simulink model "pcssp_KMAG"  (R2021b)
settings: configuration reference "configurationSettings" (kept outside this file)
model workspace (MAT data in the model file):
  D = Simulink.Parameter
  D.Value = [1; 1; 1; 1; 1; 1; 1; 1; 1; 1]
  D.DataType = 'auto'
  D.Complexity = 'real'
  D.Dimensions = [10 1]
  I = Simulink.Parameter
  I.Value = [0; 0; 0; 0; 0; 0; 0; 0; 0; 0]
  I.DataType = 'auto'
  I.Complexity = 'real'
  I.Dimensions = [10 1]
  Ke = Simulink.Parameter
  Ke.Value = [-28670  34910  -109600  -61980  15820  1380  -79930  5000  -33750  107970; -4300  49190  266010  -320680  -89150  -14470  213760  -294110  141230  -69990; -8230  89070  -109150  128070  -98530  23030  -80450  198760  -447440  298310; 60280  -203200  325320  92860  19480  -28160  246550  -127230  418190  -542920; 27220  -53430  89760  38240  33040  -9510  58170  -41770  149520  -165290; -64820  62380  -448030  96250  75680  20610  -335880  248860  -252220  351720; -79530  20450  -526450  190300  68090  33330  -374430  359300  -304180  362660; -14110  -195650  264260  12300  -144100  28740  302600  -17230  198910  -331740; 31190  108560  160080  -115050  -57970  36320  136890  -80820  -59420  128610; 16680  216660  -299770  45470  127150  30260  -279790  136410  -267230  459950; 35820  72090  -113700  76140  123830  5400  -131940  47420  -1940  106630]
  Ke.DataType = 'auto'
  Ke.Complexity = 'real'
  Ke.Dimensions = [11 10]
  N = Simulink.Parameter
  N.Value = [100; 100; 100; 100; 100; 100; 100; 100; 100; 100]
  N.DataType = 'auto'
  N.Complexity = 'real'
  N.Dimensions = [10 1]
  P = Simulink.Parameter
  P.Value = [1; 1; 1; 1; 1; 1; 1; 1; 1; 1]
  P.DataType = 'auto'
  P.Complexity = 'real'
  P.Dimensions = [10 1]
values from neighbouring files (symbols this model uses):
  D = Simulink.Parameter(ones(10,1))    [pcssp_KMAG_load_D.m]
  I = Simulink.Parameter(zeros(10,1))    [pcssp_KMAG_load_I.m]
  Ke = Simulink.Parameter(Ketemp)    [pcssp_KMAG_load_Ke.m]
  N = Simulink.Parameter(100*ones(10,1))    [pcssp_KMAG_load_N.m]
  P = Simulink.Parameter(ones(10,1))    [pcssp_KMAG_load_P.m]
  pcssp_KMAG_fp = 0.0    [pcssp_KMAG.sldd]
undefined symbols (not defined in the file or in its folder): DiscIntNeverNeededParam
settings Model: DataDictionary=pcssp_KMAG.sldd  Creator=ravenst1  LastModifiedBy=ravenst1
settings ConfigSetRef: SourceName=configurationSettings

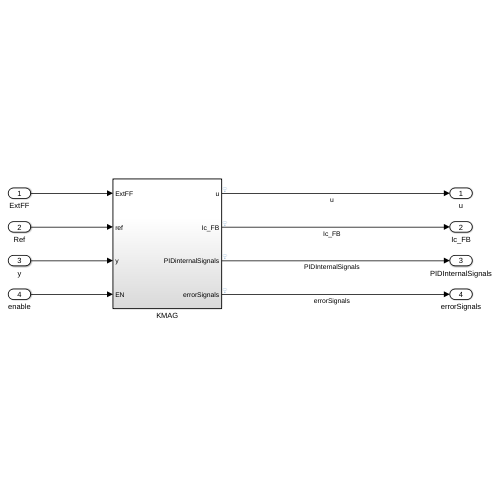
[thumbnail: Simulink's stored preview of the top-level diagram]
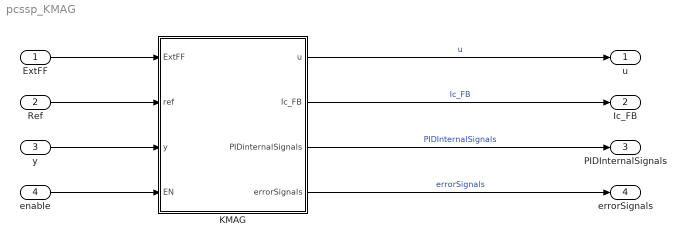
== system pcssp_KMAG ==
  ExtFF : Inport  PortDimensions=size.extFF
  Ref : Inport  Port=2  PortDimensions=size.Ref
  y : Inport  Port=3  PortDimensions=size.y
  enable : Inport  Port=4  OutDataTypeStr=double  PortDimensions=size.enable
  KMAG : Subsystem
  u : Outport
  Ic_FB : Outport  Port=2
  PIDInternalSignals : Outport  Port=3
  errorSignals : Outport  Port=4
  wires:
  KMAG/1(u) -> u/1  "u"
  KMAG/4(errorSignals) -> errorSignals/1  "errorSignals"
  KMAG/3(PIDinternalSignals) -> PIDInternalSignals/1  "PIDInternalSignals"
  KMAG/2(Ic_FB) -> Ic_FB/1  "Ic_FB"
  enable/1 -> KMAG/4(EN)
  ExtFF/1 -> KMAG/1(ExtFF)
  Ref/1 -> KMAG/2(ref)
  y/1 -> KMAG/3(y)

== system pcssp_KMAG/KMAG ==
  ExtFF : Inport
  ref : Inport  Port=2
  y : Inport  Port=3
  EN : Inport  Port=4
  "Enabled PID Block with Enabled Integration (10x10) " : Subsystem
  Ke : Constant  Value=Ke
  Logical Operator : Logic  Operator=NOT  AllPortsSameDT=off  OutDataTypeStr=boolean
  Multiply1 : Product  Inputs=**  Multiplication=Matrix(*)
  Sum : Sum  Inputs=|+-
  Sum1 : Sum  Inputs=++|
  Switch : Switch  Criteria=u2 > Threshold
  ones(10,1) : Constant  Value=1*ones(10,1)
  zeros(10,1) : Constant  Value=0
  u : Outport  PortDimensions=size.extFF
  Ic_FB : Outport  Port=2
  PIDinternalSignals : Outport  Port=3
  errorSignals : Outport  Port=4
  wires:
  "Enabled PID Block with Enabled Integration (10x10) "/1(u) -> Multiply1/2
  Sum1/1 -> Switch/3
  Logical Operator/1 -> Switch/2
  zeros(10,1)/1 -> "Enabled PID Block with Enabled Integration (10x10) "/3(Rs)
  Ke/1 -> Multiply1/1
  Sum/1 -> errorSignals/1, "Enabled PID Block with Enabled Integration (10x10) "/1(e)
  ExtFF/1 -> Sum1/1, Switch/1
  "Enabled PID Block with Enabled Integration (10x10) "/2(PIDinternalSignals) -> PIDinternalSignals/1
  ones(10,1)/1 -> "Enabled PID Block with Enabled Integration (10x10) "/2(IES)
  EN/1 -> Logical Operator/1, "Enabled PID Block with Enabled Integration (10x10) "/Enable
  ref/1 -> Sum/1
  Multiply1/1 -> Sum1/2, Ic_FB/1
  Switch/1 -> u/1
  y/1 -> Sum/2

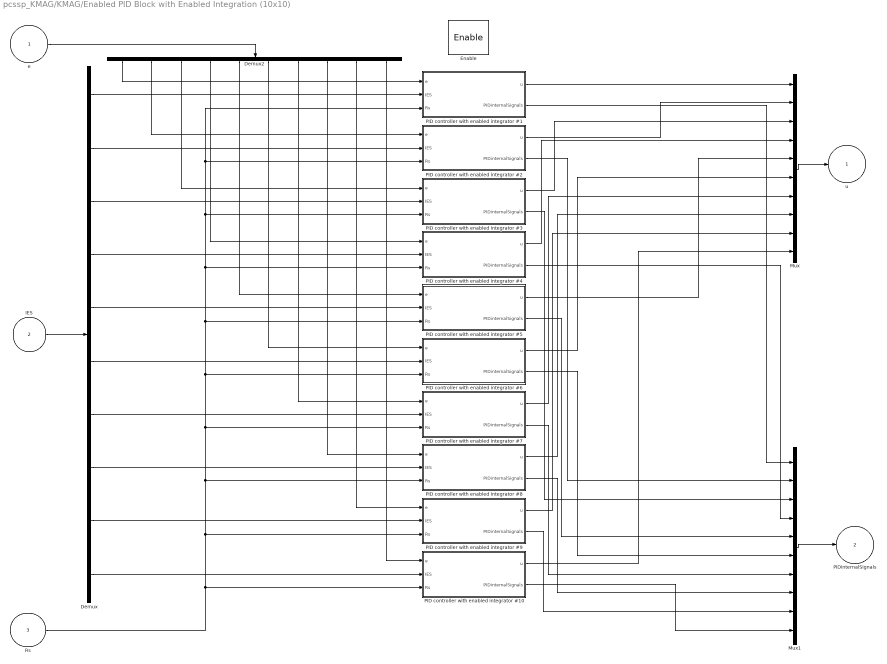
== system pcssp_KMAG/KMAG/Enabled PID Block with Enabled Integration (10x10)  ==
  e : Inport
  IES : Inport  Port=2
  Rs : Inport  Port=3
  Enable : EnablePort  StatesWhenEnabling=reset
  Demux : Demux  Outputs=10
  Demux2 : Demux  Outputs=10
  Mux : Mux  Inputs=10
  Mux1 : Mux  Inputs=10
  PID controller with enabled integrator #1 : Subsystem
  PID controller with enabled integrator #10 : Subsystem
  PID controller with enabled integrator #2 : Subsystem
  PID controller with enabled integrator #3 : Subsystem
  PID controller with enabled integrator #4 : Subsystem
  PID controller with enabled integrator #5 : Subsystem
  PID controller with enabled integrator #6 : Subsystem
  PID controller with enabled integrator #7 : Subsystem
  PID controller with enabled integrator #8 : Subsystem
  PID controller with enabled integrator #9 : Subsystem
  u : Outport
  PIDinternalSignals : Outport  Port=2
  wires:
  e/1 -> Demux2/1
  IES/1 -> Demux/1
  PID controller with enabled integrator #5/2(PIDinternalSignals) -> Mux1/5
  PID controller with enabled integrator #4/2(PIDinternalSignals) -> Mux1/4
  PID controller with enabled integrator #3/2(PIDinternalSignals) -> Mux1/3
  PID controller with enabled integrator #2/2(PIDinternalSignals) -> Mux1/2
  PID controller with enabled integrator #1/2(PIDinternalSignals) -> Mux1/1
  PID controller with enabled integrator #6/2(PIDinternalSignals) -> Mux1/6
  PID controller with enabled integrator #7/2(PIDinternalSignals) -> Mux1/7
  PID controller with enabled integrator #8/2(PIDinternalSignals) -> Mux1/8
  PID controller with enabled integrator #9/2(PIDinternalSignals) -> Mux1/9
  PID controller with enabled integrator #10/2(PIDinternalSignals) -> Mux1/10
  PID controller with enabled integrator #1/1(u) -> Mux/1
  PID controller with enabled integrator #2/1(u) -> Mux/2
  PID controller with enabled integrator #3/1(u) -> Mux/3
  PID controller with enabled integrator #4/1(u) -> Mux/4
  PID controller with enabled integrator #5/1(u) -> Mux/5
  PID controller with enabled integrator #6/1(u) -> Mux/6
  PID controller with enabled integrator #7/1(u) -> Mux/7
  PID controller with enabled integrator #8/1(u) -> Mux/8
  PID controller with enabled integrator #9/1(u) -> Mux/9
  PID controller with enabled integrator #10/1(u) -> Mux/10
  Mux1/1 -> PIDinternalSignals/1
  Demux/4 -> PID controller with enabled integrator #4/2(IES)
  Demux2/9 -> PID controller with enabled integrator #9/1(e)
  Demux/7 -> PID controller with enabled integrator #7/2(IES)
  Rs/1 -> PID controller with enabled integrator #10/3(Rs), PID controller with enabled integrator #9/3(Rs), PID controller with enabled integrator #8/3(Rs), PID controller with enabled integrator #7/3(Rs), PID controller with enabled integrator #6/3(Rs), PID controller with enabled integrator #5/3(Rs), PID controller with enabled integrator #4/3(Rs), PID controller with enabled integrator #3/3(Rs), PID controller with enabled integrator #2/3(Rs), PID controller with enabled integrator #1/3(Rs)
  Demux/1 -> PID controller with enabled integrator #1/2(IES)
  Demux/5 -> PID controller with enabled integrator #5/2(IES)
  Demux/6 -> PID controller with enabled integrator #6/2(IES)
  Demux/2 -> PID controller with enabled integrator #2/2(IES)
  Demux/8 -> PID controller with enabled integrator #8/2(IES)
  Demux/10 -> PID controller with enabled integrator #10/2(IES)
  Demux2/10 -> PID controller with enabled integrator #10/1(e)
  Demux2/4 -> PID controller with enabled integrator #4/1(e)
  Demux2/3 -> PID controller with enabled integrator #3/1(e)
  Demux2/2 -> PID controller with enabled integrator #2/1(e)
  Demux/3 -> PID controller with enabled integrator #3/2(IES)
  Demux2/5 -> PID controller with enabled integrator #5/1(e)
  Mux/1 -> u/1
  Demux2/8 -> PID controller with enabled integrator #8/1(e)
  Demux2/7 -> PID controller with enabled integrator #7/1(e)
  Demux2/6 -> PID controller with enabled integrator #6/1(e)
  Demux/9 -> PID controller with enabled integrator #9/2(IES)
  Demux2/1 -> PID controller with enabled integrator #1/1(e)

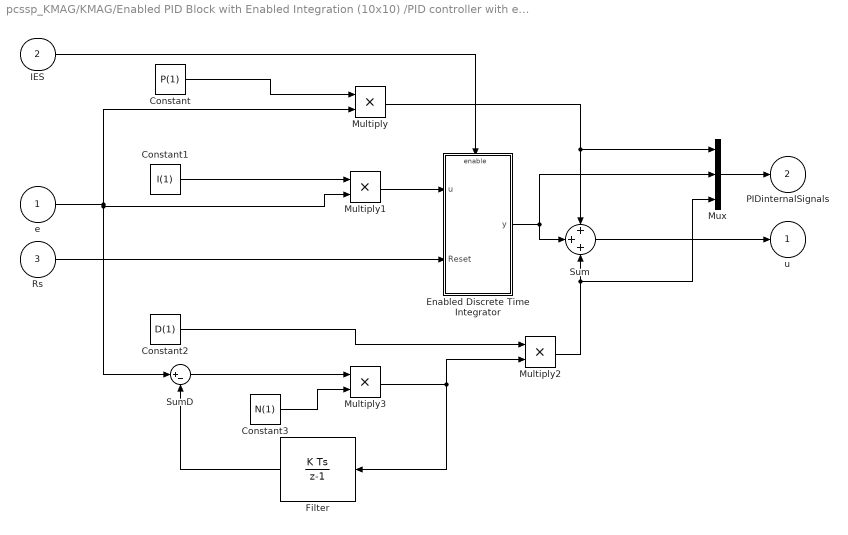
== system pcssp_KMAG/KMAG/Enabled PID Block with Enabled Integration (10x10) /PID controller with enabled integrator #1 ==
  e : Inport
  IES : Inport  Port=2
  Rs : Inport  Port=3
  Constant : Constant  Value=P(1)
  Constant1 : Constant  Value=I(1)
  Constant2 : Constant  Value=D(1)
  Constant3 : Constant  Value=N(1)
  Enabled Discrete Time Integrator : Subsystem
  Filter : DiscreteIntegrator  DisableCoverage=on  SampleTime=pcssp_KMAG_fp.timing.dt  ICPrevOutput=DiscIntNeverNeededParam  ICPrevScaledInput=DiscIntNeverNeededParam
  Multiply{,1..3} (4 alike) : Product  Inputs=**
  Mux : Mux  Inputs=3
  Sum : Sum  Inputs=+++
  SumD : Sum  DisableCoverage=on  Inputs=|+-
  u : Outport  InitialOutput=0
  PIDinternalSignals : Outport  Port=2  InitialOutput=0
  wires:
  Multiply1/1 -> Enabled Discrete Time Integrator/1(u)
  Filter/1 -> SumD/2
  Enabled Discrete Time Integrator/1(y) -> Mux/2, Sum/2
  IES/1 -> Enabled Discrete Time Integrator/Enable
  Sum/1 -> u/1
  Multiply/1 -> Sum/1, Mux/1
  e/1 -> Multiply/2, Multiply1/2, SumD/1
  Rs/1 -> Enabled Discrete Time Integrator/2(Reset)
  Mux/1 -> PIDinternalSignals/1
  Constant/1 -> Multiply/1
  Multiply3/1 -> Multiply2/2, Filter/1
  Constant2/1 -> Multiply2/1
  Multiply2/1 -> Sum/3, Mux/3
  Constant3/1 -> Multiply3/2
  SumD/1 -> Multiply3/1
  Constant1/1 -> Multiply1/1

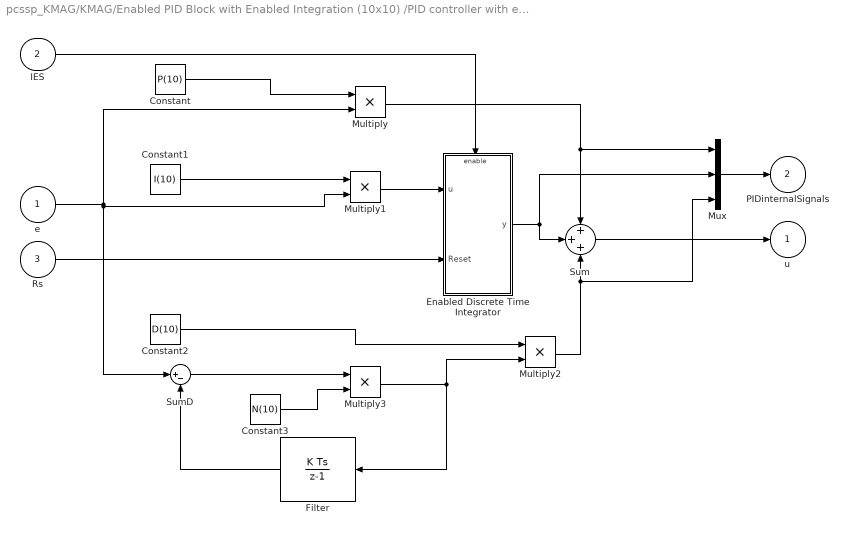
== system pcssp_KMAG/KMAG/Enabled PID Block with Enabled Integration (10x10) /PID controller with enabled integrator #10 ==
  e : Inport
  IES : Inport  Port=2
  Rs : Inport  Port=3
  Constant : Constant  Value=P(10)
  Constant1 : Constant  Value=I(10)
  Constant2 : Constant  Value=D(10)
  Constant3 : Constant  Value=N(10)
  Enabled Discrete Time Integrator : Subsystem
  Filter : DiscreteIntegrator  DisableCoverage=on  SampleTime=pcssp_KMAG_fp.timing.dt  ICPrevOutput=DiscIntNeverNeededParam  ICPrevScaledInput=DiscIntNeverNeededParam
  Multiply{,1..3} (4 alike) : Product  Inputs=**
  Mux : Mux  Inputs=3
  Sum : Sum  Inputs=+++
  SumD : Sum  DisableCoverage=on  Inputs=|+-
  u : Outport  InitialOutput=0
  PIDinternalSignals : Outport  Port=2  InitialOutput=0
  wires:
  Multiply1/1 -> Enabled Discrete Time Integrator/1(u)
  Filter/1 -> SumD/2
  Enabled Discrete Time Integrator/1(y) -> Mux/2, Sum/2
  IES/1 -> Enabled Discrete Time Integrator/Enable
  Sum/1 -> u/1
  Multiply/1 -> Sum/1, Mux/1
  e/1 -> Multiply/2, Multiply1/2, SumD/1
  Rs/1 -> Enabled Discrete Time Integrator/2(Reset)
  Mux/1 -> PIDinternalSignals/1
  Constant/1 -> Multiply/1
  Multiply3/1 -> Multiply2/2, Filter/1
  Constant2/1 -> Multiply2/1
  Multiply2/1 -> Sum/3, Mux/3
  Constant3/1 -> Multiply3/2
  SumD/1 -> Multiply3/1
  Constant1/1 -> Multiply1/1

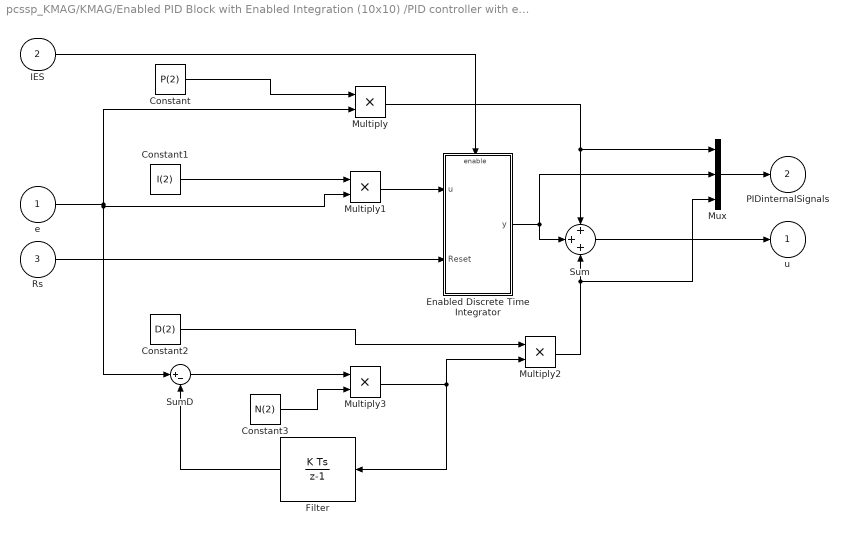
== system pcssp_KMAG/KMAG/Enabled PID Block with Enabled Integration (10x10) /PID controller with enabled integrator #2 ==
  e : Inport
  IES : Inport  Port=2
  Rs : Inport  Port=3
  Constant : Constant  Value=P(2)
  Constant1 : Constant  Value=I(2)
  Constant2 : Constant  Value=D(2)
  Constant3 : Constant  Value=N(2)
  Enabled Discrete Time Integrator : Subsystem
  Filter : DiscreteIntegrator  DisableCoverage=on  SampleTime=pcssp_KMAG_fp.timing.dt  ICPrevOutput=DiscIntNeverNeededParam  ICPrevScaledInput=DiscIntNeverNeededParam
  Multiply{,1..3} (4 alike) : Product  Inputs=**
  Mux : Mux  Inputs=3
  Sum : Sum  Inputs=+++
  SumD : Sum  DisableCoverage=on  Inputs=|+-
  u : Outport  InitialOutput=0
  PIDinternalSignals : Outport  Port=2  InitialOutput=0
  wires:
  Multiply1/1 -> Enabled Discrete Time Integrator/1(u)
  Filter/1 -> SumD/2
  Enabled Discrete Time Integrator/1(y) -> Mux/2, Sum/2
  IES/1 -> Enabled Discrete Time Integrator/Enable
  Sum/1 -> u/1
  Multiply/1 -> Sum/1, Mux/1
  e/1 -> Multiply/2, Multiply1/2, SumD/1
  Rs/1 -> Enabled Discrete Time Integrator/2(Reset)
  Mux/1 -> PIDinternalSignals/1
  Constant/1 -> Multiply/1
  Multiply3/1 -> Multiply2/2, Filter/1
  Constant2/1 -> Multiply2/1
  Multiply2/1 -> Sum/3, Mux/3
  Constant3/1 -> Multiply3/2
  SumD/1 -> Multiply3/1
  Constant1/1 -> Multiply1/1

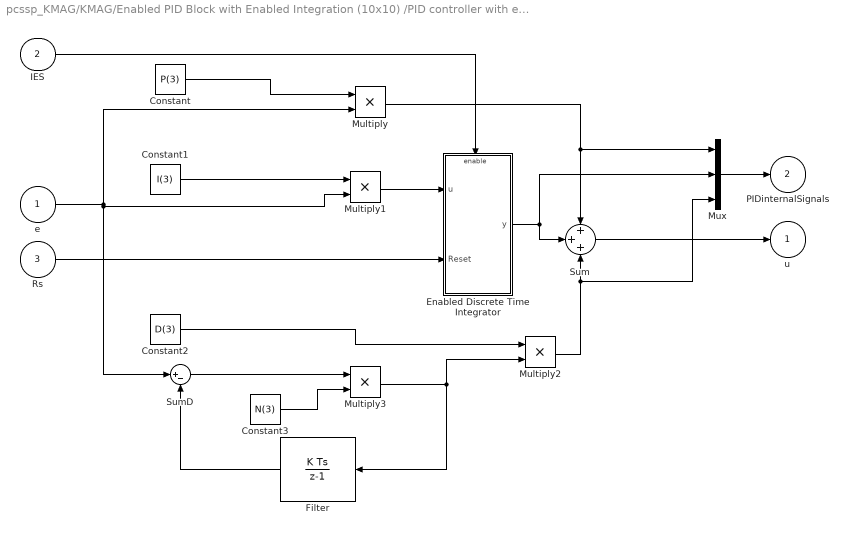
== system pcssp_KMAG/KMAG/Enabled PID Block with Enabled Integration (10x10) /PID controller with enabled integrator #3 ==
  e : Inport
  IES : Inport  Port=2
  Rs : Inport  Port=3
  Constant : Constant  Value=P(3)
  Constant1 : Constant  Value=I(3)
  Constant2 : Constant  Value=D(3)
  Constant3 : Constant  Value=N(3)
  Enabled Discrete Time Integrator : Subsystem
  Filter : DiscreteIntegrator  DisableCoverage=on  SampleTime=pcssp_KMAG_fp.timing.dt  ICPrevOutput=DiscIntNeverNeededParam  ICPrevScaledInput=DiscIntNeverNeededParam
  Multiply{,1..3} (4 alike) : Product  Inputs=**
  Mux : Mux  Inputs=3
  Sum : Sum  Inputs=+++
  SumD : Sum  DisableCoverage=on  Inputs=|+-
  u : Outport  InitialOutput=0
  PIDinternalSignals : Outport  Port=2  InitialOutput=0
  wires:
  Multiply1/1 -> Enabled Discrete Time Integrator/1(u)
  Filter/1 -> SumD/2
  Enabled Discrete Time Integrator/1(y) -> Mux/2, Sum/2
  IES/1 -> Enabled Discrete Time Integrator/Enable
  Sum/1 -> u/1
  Multiply/1 -> Sum/1, Mux/1
  e/1 -> Multiply/2, Multiply1/2, SumD/1
  Rs/1 -> Enabled Discrete Time Integrator/2(Reset)
  Mux/1 -> PIDinternalSignals/1
  Constant/1 -> Multiply/1
  Multiply3/1 -> Multiply2/2, Filter/1
  Constant2/1 -> Multiply2/1
  Multiply2/1 -> Sum/3, Mux/3
  Constant3/1 -> Multiply3/2
  SumD/1 -> Multiply3/1
  Constant1/1 -> Multiply1/1

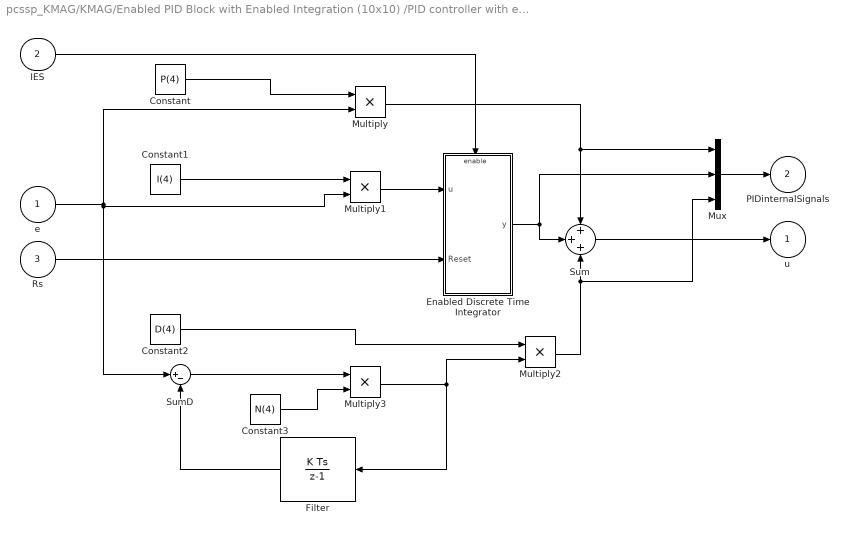
== system pcssp_KMAG/KMAG/Enabled PID Block with Enabled Integration (10x10) /PID controller with enabled integrator #4 ==
  e : Inport
  IES : Inport  Port=2
  Rs : Inport  Port=3
  Constant : Constant  Value=P(4)
  Constant1 : Constant  Value=I(4)
  Constant2 : Constant  Value=D(4)
  Constant3 : Constant  Value=N(4)
  Enabled Discrete Time Integrator : Subsystem
  Filter : DiscreteIntegrator  DisableCoverage=on  SampleTime=pcssp_KMAG_fp.timing.dt  ICPrevOutput=DiscIntNeverNeededParam  ICPrevScaledInput=DiscIntNeverNeededParam
  Multiply{,1..3} (4 alike) : Product  Inputs=**
  Mux : Mux  Inputs=3
  Sum : Sum  Inputs=+++
  SumD : Sum  DisableCoverage=on  Inputs=|+-
  u : Outport  InitialOutput=0
  PIDinternalSignals : Outport  Port=2  InitialOutput=0
  wires:
  Multiply1/1 -> Enabled Discrete Time Integrator/1(u)
  Filter/1 -> SumD/2
  Enabled Discrete Time Integrator/1(y) -> Mux/2, Sum/2
  IES/1 -> Enabled Discrete Time Integrator/Enable
  Sum/1 -> u/1
  Multiply/1 -> Sum/1, Mux/1
  e/1 -> Multiply/2, Multiply1/2, SumD/1
  Rs/1 -> Enabled Discrete Time Integrator/2(Reset)
  Mux/1 -> PIDinternalSignals/1
  Constant/1 -> Multiply/1
  Multiply3/1 -> Multiply2/2, Filter/1
  Constant2/1 -> Multiply2/1
  Multiply2/1 -> Sum/3, Mux/3
  Constant3/1 -> Multiply3/2
  SumD/1 -> Multiply3/1
  Constant1/1 -> Multiply1/1

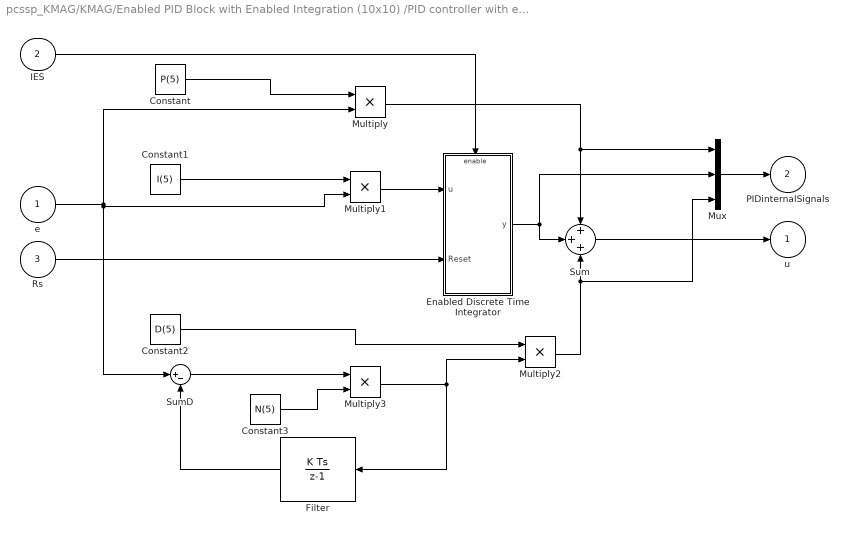
== system pcssp_KMAG/KMAG/Enabled PID Block with Enabled Integration (10x10) /PID controller with enabled integrator #5 ==
  e : Inport
  IES : Inport  Port=2
  Rs : Inport  Port=3
  Constant : Constant  Value=P(5)
  Constant1 : Constant  Value=I(5)
  Constant2 : Constant  Value=D(5)
  Constant3 : Constant  Value=N(5)
  Enabled Discrete Time Integrator : Subsystem
  Filter : DiscreteIntegrator  DisableCoverage=on  SampleTime=pcssp_KMAG_fp.timing.dt  ICPrevOutput=DiscIntNeverNeededParam  ICPrevScaledInput=DiscIntNeverNeededParam
  Multiply{,1..3} (4 alike) : Product  Inputs=**
  Mux : Mux  Inputs=3
  Sum : Sum  Inputs=+++
  SumD : Sum  DisableCoverage=on  Inputs=|+-
  u : Outport  InitialOutput=0
  PIDinternalSignals : Outport  Port=2  InitialOutput=0
  wires:
  Multiply1/1 -> Enabled Discrete Time Integrator/1(u)
  Filter/1 -> SumD/2
  Enabled Discrete Time Integrator/1(y) -> Mux/2, Sum/2
  IES/1 -> Enabled Discrete Time Integrator/Enable
  Sum/1 -> u/1
  Multiply/1 -> Sum/1, Mux/1
  e/1 -> Multiply/2, Multiply1/2, SumD/1
  Rs/1 -> Enabled Discrete Time Integrator/2(Reset)
  Mux/1 -> PIDinternalSignals/1
  Constant/1 -> Multiply/1
  Multiply3/1 -> Multiply2/2, Filter/1
  Constant2/1 -> Multiply2/1
  Multiply2/1 -> Sum/3, Mux/3
  Constant3/1 -> Multiply3/2
  SumD/1 -> Multiply3/1
  Constant1/1 -> Multiply1/1

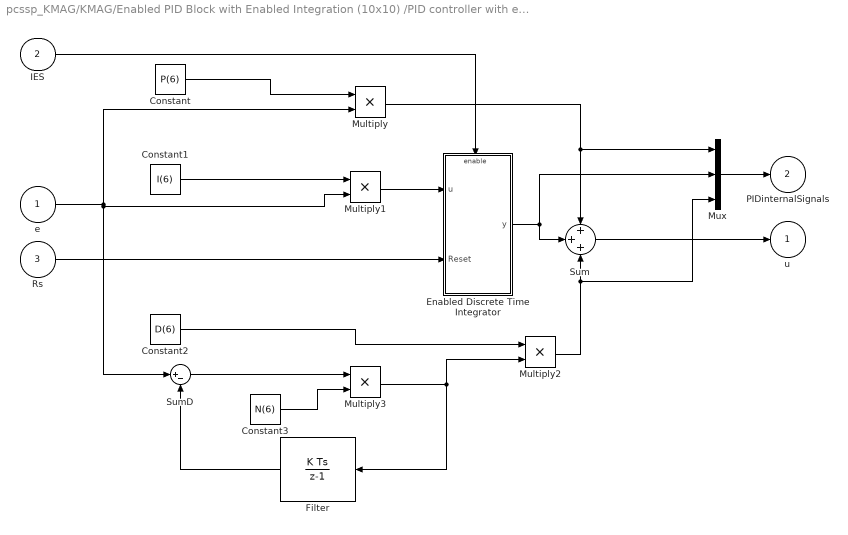
== system pcssp_KMAG/KMAG/Enabled PID Block with Enabled Integration (10x10) /PID controller with enabled integrator #6 ==
  e : Inport
  IES : Inport  Port=2
  Rs : Inport  Port=3
  Constant : Constant  Value=P(6)
  Constant1 : Constant  Value=I(6)
  Constant2 : Constant  Value=D(6)
  Constant3 : Constant  Value=N(6)
  Enabled Discrete Time Integrator : Subsystem
  Filter : DiscreteIntegrator  DisableCoverage=on  SampleTime=pcssp_KMAG_fp.timing.dt  ICPrevOutput=DiscIntNeverNeededParam  ICPrevScaledInput=DiscIntNeverNeededParam
  Multiply{,1..3} (4 alike) : Product  Inputs=**
  Mux : Mux  Inputs=3
  Sum : Sum  Inputs=+++
  SumD : Sum  DisableCoverage=on  Inputs=|+-
  u : Outport  InitialOutput=0
  PIDinternalSignals : Outport  Port=2  InitialOutput=0
  wires:
  Multiply1/1 -> Enabled Discrete Time Integrator/1(u)
  Filter/1 -> SumD/2
  Enabled Discrete Time Integrator/1(y) -> Mux/2, Sum/2
  IES/1 -> Enabled Discrete Time Integrator/Enable
  Sum/1 -> u/1
  Multiply/1 -> Sum/1, Mux/1
  e/1 -> Multiply/2, Multiply1/2, SumD/1
  Rs/1 -> Enabled Discrete Time Integrator/2(Reset)
  Mux/1 -> PIDinternalSignals/1
  Constant/1 -> Multiply/1
  Multiply3/1 -> Multiply2/2, Filter/1
  Constant2/1 -> Multiply2/1
  Multiply2/1 -> Sum/3, Mux/3
  Constant3/1 -> Multiply3/2
  SumD/1 -> Multiply3/1
  Constant1/1 -> Multiply1/1

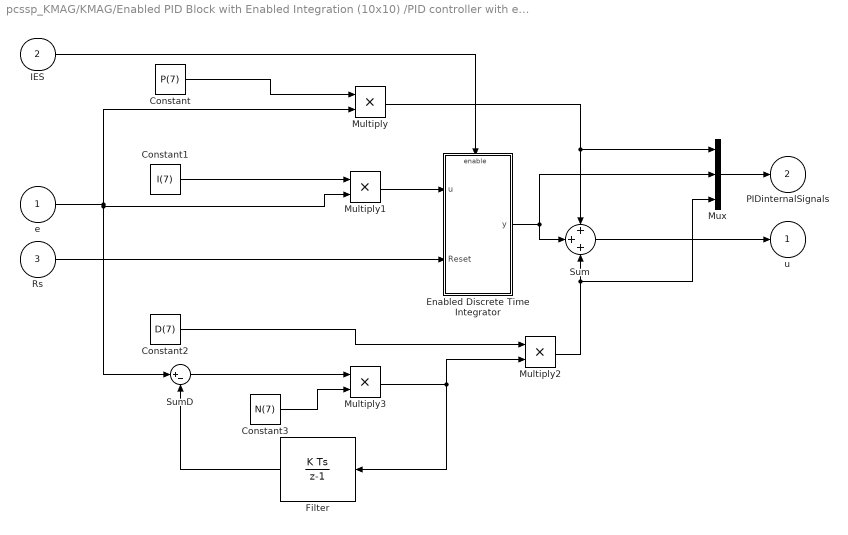
== system pcssp_KMAG/KMAG/Enabled PID Block with Enabled Integration (10x10) /PID controller with enabled integrator #7 ==
  e : Inport
  IES : Inport  Port=2
  Rs : Inport  Port=3
  Constant : Constant  Value=P(7)
  Constant1 : Constant  Value=I(7)
  Constant2 : Constant  Value=D(7)
  Constant3 : Constant  Value=N(7)
  Enabled Discrete Time Integrator : Subsystem
  Filter : DiscreteIntegrator  DisableCoverage=on  SampleTime=pcssp_KMAG_fp.timing.dt  ICPrevOutput=DiscIntNeverNeededParam  ICPrevScaledInput=DiscIntNeverNeededParam
  Multiply{,1..3} (4 alike) : Product  Inputs=**
  Mux : Mux  Inputs=3
  Sum : Sum  Inputs=+++
  SumD : Sum  DisableCoverage=on  Inputs=|+-
  u : Outport  InitialOutput=0
  PIDinternalSignals : Outport  Port=2  InitialOutput=0
  wires:
  Multiply1/1 -> Enabled Discrete Time Integrator/1(u)
  Filter/1 -> SumD/2
  Enabled Discrete Time Integrator/1(y) -> Mux/2, Sum/2
  IES/1 -> Enabled Discrete Time Integrator/Enable
  Sum/1 -> u/1
  Multiply/1 -> Sum/1, Mux/1
  e/1 -> Multiply/2, Multiply1/2, SumD/1
  Rs/1 -> Enabled Discrete Time Integrator/2(Reset)
  Mux/1 -> PIDinternalSignals/1
  Constant/1 -> Multiply/1
  Multiply3/1 -> Multiply2/2, Filter/1
  Constant2/1 -> Multiply2/1
  Multiply2/1 -> Sum/3, Mux/3
  Constant3/1 -> Multiply3/2
  SumD/1 -> Multiply3/1
  Constant1/1 -> Multiply1/1

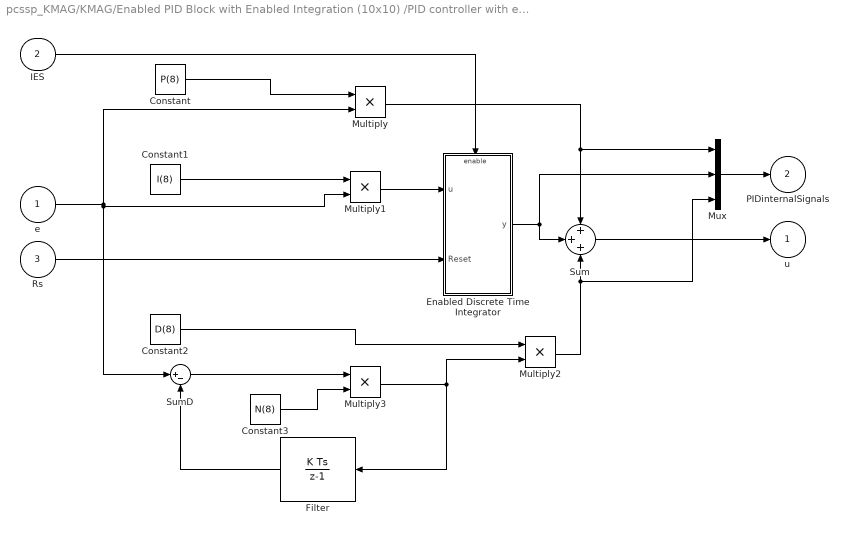
== system pcssp_KMAG/KMAG/Enabled PID Block with Enabled Integration (10x10) /PID controller with enabled integrator #8 ==
  e : Inport
  IES : Inport  Port=2
  Rs : Inport  Port=3
  Constant : Constant  Value=P(8)
  Constant1 : Constant  Value=I(8)
  Constant2 : Constant  Value=D(8)
  Constant3 : Constant  Value=N(8)
  Enabled Discrete Time Integrator : Subsystem
  Filter : DiscreteIntegrator  DisableCoverage=on  SampleTime=pcssp_KMAG_fp.timing.dt  ICPrevOutput=DiscIntNeverNeededParam  ICPrevScaledInput=DiscIntNeverNeededParam
  Multiply{,1..3} (4 alike) : Product  Inputs=**
  Mux : Mux  Inputs=3
  Sum : Sum  Inputs=+++
  SumD : Sum  DisableCoverage=on  Inputs=|+-
  u : Outport  InitialOutput=0
  PIDinternalSignals : Outport  Port=2  InitialOutput=0
  wires:
  Multiply1/1 -> Enabled Discrete Time Integrator/1(u)
  Filter/1 -> SumD/2
  Enabled Discrete Time Integrator/1(y) -> Mux/2, Sum/2
  IES/1 -> Enabled Discrete Time Integrator/Enable
  Sum/1 -> u/1
  Multiply/1 -> Sum/1, Mux/1
  e/1 -> Multiply/2, Multiply1/2, SumD/1
  Rs/1 -> Enabled Discrete Time Integrator/2(Reset)
  Mux/1 -> PIDinternalSignals/1
  Constant/1 -> Multiply/1
  Multiply3/1 -> Multiply2/2, Filter/1
  Constant2/1 -> Multiply2/1
  Multiply2/1 -> Sum/3, Mux/3
  Constant3/1 -> Multiply3/2
  SumD/1 -> Multiply3/1
  Constant1/1 -> Multiply1/1

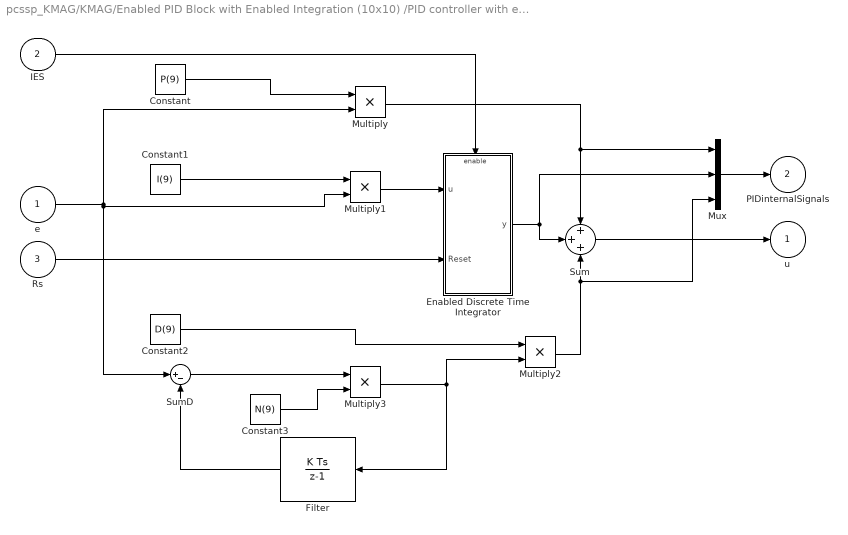
== system pcssp_KMAG/KMAG/Enabled PID Block with Enabled Integration (10x10) /PID controller with enabled integrator #9 ==
  e : Inport
  IES : Inport  Port=2
  Rs : Inport  Port=3
  Constant : Constant  Value=P(9)
  Constant1 : Constant  Value=I(9)
  Constant2 : Constant  Value=D(9)
  Constant3 : Constant  Value=N(9)
  Enabled Discrete Time Integrator : Subsystem
  Filter : DiscreteIntegrator  DisableCoverage=on  SampleTime=pcssp_KMAG_fp.timing.dt  ICPrevOutput=DiscIntNeverNeededParam  ICPrevScaledInput=DiscIntNeverNeededParam
  Multiply{,1..3} (4 alike) : Product  Inputs=**
  Mux : Mux  Inputs=3
  Sum : Sum  Inputs=+++
  SumD : Sum  DisableCoverage=on  Inputs=|+-
  u : Outport  InitialOutput=0
  PIDinternalSignals : Outport  Port=2  InitialOutput=0
  wires:
  Multiply1/1 -> Enabled Discrete Time Integrator/1(u)
  Filter/1 -> SumD/2
  Enabled Discrete Time Integrator/1(y) -> Mux/2, Sum/2
  IES/1 -> Enabled Discrete Time Integrator/Enable
  Sum/1 -> u/1
  Multiply/1 -> Sum/1, Mux/1
  e/1 -> Multiply/2, Multiply1/2, SumD/1
  Rs/1 -> Enabled Discrete Time Integrator/2(Reset)
  Mux/1 -> PIDinternalSignals/1
  Constant/1 -> Multiply/1
  Multiply3/1 -> Multiply2/2, Filter/1
  Constant2/1 -> Multiply2/1
  Multiply2/1 -> Sum/3, Mux/3
  Constant3/1 -> Multiply3/2
  SumD/1 -> Multiply3/1
  Constant1/1 -> Multiply1/1

== system pcssp_KMAG/KMAG/Enabled PID Block with Enabled Integration (10x10) /PID controller with enabled integrator #1/Enabled Discrete Time Integrator ==
  u : Inport
  Reset : Inport  Port=2
  Enable : EnablePort
  Filter : DiscreteIntegrator  DisableCoverage=on  ExternalReset=rising  SampleTime=pcssp_KMAG_fp.timing.dt  ICPrevOutput=DiscIntNeverNeededParam  ICPrevScaledInput=DiscIntNeverNeededParam
  y : Outport
  wires:
  Reset/1 -> Filter/2
  Filter/1 -> y/1
  u/1 -> Filter/1

== system pcssp_KMAG/KMAG/Enabled PID Block with Enabled Integration (10x10) /PID controller with enabled integrator #10/Enabled Discrete Time Integrator ==
  u : Inport
  Reset : Inport  Port=2
  Enable : EnablePort
  Filter : DiscreteIntegrator  DisableCoverage=on  ExternalReset=rising  SampleTime=pcssp_KMAG_fp.timing.dt  ICPrevOutput=DiscIntNeverNeededParam  ICPrevScaledInput=DiscIntNeverNeededParam
  y : Outport
  wires:
  Reset/1 -> Filter/2
  Filter/1 -> y/1
  u/1 -> Filter/1

== system pcssp_KMAG/KMAG/Enabled PID Block with Enabled Integration (10x10) /PID controller with enabled integrator #2/Enabled Discrete Time Integrator ==
  u : Inport
  Reset : Inport  Port=2
  Enable : EnablePort
  Filter : DiscreteIntegrator  DisableCoverage=on  ExternalReset=rising  SampleTime=pcssp_KMAG_fp.timing.dt  ICPrevOutput=DiscIntNeverNeededParam  ICPrevScaledInput=DiscIntNeverNeededParam
  y : Outport
  wires:
  Reset/1 -> Filter/2
  Filter/1 -> y/1
  u/1 -> Filter/1

== system pcssp_KMAG/KMAG/Enabled PID Block with Enabled Integration (10x10) /PID controller with enabled integrator #3/Enabled Discrete Time Integrator ==
  u : Inport
  Reset : Inport  Port=2
  Enable : EnablePort
  Filter : DiscreteIntegrator  DisableCoverage=on  ExternalReset=rising  SampleTime=pcssp_KMAG_fp.timing.dt  ICPrevOutput=DiscIntNeverNeededParam  ICPrevScaledInput=DiscIntNeverNeededParam
  y : Outport
  wires:
  Reset/1 -> Filter/2
  Filter/1 -> y/1
  u/1 -> Filter/1

== system pcssp_KMAG/KMAG/Enabled PID Block with Enabled Integration (10x10) /PID controller with enabled integrator #4/Enabled Discrete Time Integrator ==
  u : Inport
  Reset : Inport  Port=2
  Enable : EnablePort
  Filter : DiscreteIntegrator  DisableCoverage=on  ExternalReset=rising  SampleTime=pcssp_KMAG_fp.timing.dt  ICPrevOutput=DiscIntNeverNeededParam  ICPrevScaledInput=DiscIntNeverNeededParam
  y : Outport
  wires:
  Reset/1 -> Filter/2
  Filter/1 -> y/1
  u/1 -> Filter/1

== system pcssp_KMAG/KMAG/Enabled PID Block with Enabled Integration (10x10) /PID controller with enabled integrator #5/Enabled Discrete Time Integrator ==
  u : Inport
  Reset : Inport  Port=2
  Enable : EnablePort
  Filter : DiscreteIntegrator  DisableCoverage=on  ExternalReset=rising  SampleTime=pcssp_KMAG_fp.timing.dt  ICPrevOutput=DiscIntNeverNeededParam  ICPrevScaledInput=DiscIntNeverNeededParam
  y : Outport
  wires:
  Reset/1 -> Filter/2
  Filter/1 -> y/1
  u/1 -> Filter/1

== system pcssp_KMAG/KMAG/Enabled PID Block with Enabled Integration (10x10) /PID controller with enabled integrator #6/Enabled Discrete Time Integrator ==
  u : Inport
  Reset : Inport  Port=2
  Enable : EnablePort
  Filter : DiscreteIntegrator  DisableCoverage=on  ExternalReset=rising  SampleTime=pcssp_KMAG_fp.timing.dt  ICPrevOutput=DiscIntNeverNeededParam  ICPrevScaledInput=DiscIntNeverNeededParam
  y : Outport
  wires:
  Reset/1 -> Filter/2
  Filter/1 -> y/1
  u/1 -> Filter/1

== system pcssp_KMAG/KMAG/Enabled PID Block with Enabled Integration (10x10) /PID controller with enabled integrator #7/Enabled Discrete Time Integrator ==
  u : Inport
  Reset : Inport  Port=2
  Enable : EnablePort
  Filter : DiscreteIntegrator  DisableCoverage=on  ExternalReset=rising  SampleTime=pcssp_KMAG_fp.timing.dt  ICPrevOutput=DiscIntNeverNeededParam  ICPrevScaledInput=DiscIntNeverNeededParam
  y : Outport
  wires:
  Reset/1 -> Filter/2
  Filter/1 -> y/1
  u/1 -> Filter/1

== system pcssp_KMAG/KMAG/Enabled PID Block with Enabled Integration (10x10) /PID controller with enabled integrator #8/Enabled Discrete Time Integrator ==
  u : Inport
  Reset : Inport  Port=2
  Enable : EnablePort
  Filter : DiscreteIntegrator  DisableCoverage=on  ExternalReset=rising  SampleTime=pcssp_KMAG_fp.timing.dt  ICPrevOutput=DiscIntNeverNeededParam  ICPrevScaledInput=DiscIntNeverNeededParam
  y : Outport
  wires:
  Reset/1 -> Filter/2
  Filter/1 -> y/1
  u/1 -> Filter/1

== system pcssp_KMAG/KMAG/Enabled PID Block with Enabled Integration (10x10) /PID controller with enabled integrator #9/Enabled Discrete Time Integrator ==
  u : Inport
  Reset : Inport  Port=2
  Enable : EnablePort
  Filter : DiscreteIntegrator  DisableCoverage=on  ExternalReset=rising  SampleTime=pcssp_KMAG_fp.timing.dt  ICPrevOutput=DiscIntNeverNeededParam  ICPrevScaledInput=DiscIntNeverNeededParam
  y : Outport
  wires:
  Reset/1 -> Filter/2
  Filter/1 -> y/1
  u/1 -> Filter/1
